simulink model "power_estimator2"  (R2015a)
settings: Solver=ode45  StartTime=0.0  StopTime=10.0  RelTol=1e-3
values from neighbouring files (symbols this model uses):
  L = 8e-3    (= 0.008)    [VOC_param.m]    (also in VOC_param_paper.m = 0.003; controller_parameters.m = 0.003; current_controller_param.m = 0.005; power_control_param.m = 0.01)
settings Model: Creator=rblan  LastModifiedBy=rblan

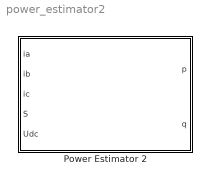
== system power_estimator2 ==
  Power Estimator 2 : Subsystem

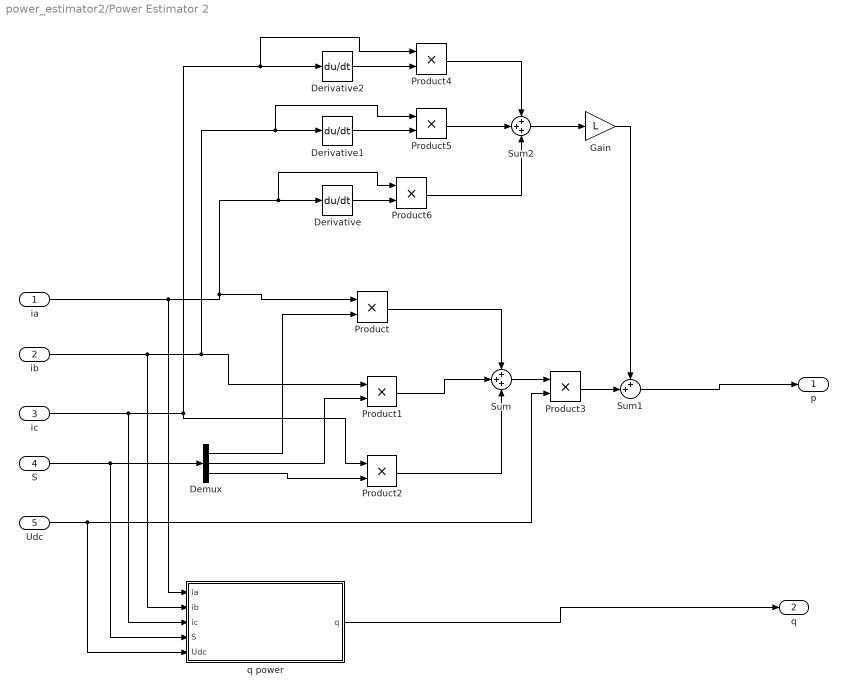
== system power_estimator2/Power Estimator 2 ==
  ia : Inport
  "ib " : Inport  Port=2
  "ic " : Inport  Port=3
  "S " : Inport  Port=4
  Udc : Inport  Port=5
  Demux : Demux  Outputs=3
  Derivative : Derivative
  Derivative1 : Derivative
  Derivative2 : Derivative
  Gain : Gain  Gain=L
  Product{,1..6} (7 alike) : Product
  Sum : Sum  Inputs=+++
  Sum1 : Sum  Inputs=++|
  Sum2 : Sum  Inputs=+++
  "q power " : Subsystem
  p : Outport
  q : Outport  Port=2
  wires:
  "S "/1 -> "q power "/4("S "), Demux/1
  Demux/1 -> Product/2
  ia/1 -> "q power "/1(ia), Product6/1, Derivative/1, Product/1
  "ib "/1 -> "q power "/2("ib "), Product5/1, Derivative1/1, Product1/1
  Demux/2 -> Product1/2
  Demux/3 -> Product2/2
  Product/1 -> Sum/1
  Product1/1 -> Sum/2
  Product2/1 -> Sum/3
  Sum/1 -> Product3/1
  Derivative2/1 -> Product4/2
  Derivative1/1 -> Product5/2
  Derivative/1 -> Product6/2
  Product4/1 -> Sum2/1
  Product5/1 -> Sum2/2
  Product6/1 -> Sum2/3
  Sum2/1 -> Gain/1
  Product3/1 -> Sum1/2
  Gain/1 -> Sum1/1
  "ic "/1 -> "q power "/3("ic "), Product2/1, Product4/1, Derivative2/1
  Udc/1 -> "q power "/5(Udc), Product3/2
  "q power "/1("q ") -> q/1
  Sum1/1 -> p/1

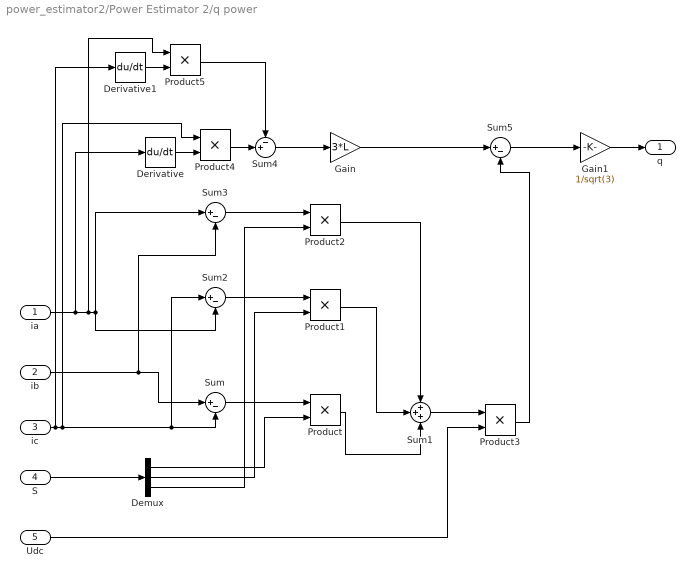
== system power_estimator2/Power Estimator 2/q power  ==
  ia : Inport
  "ib " : Inport  Port=2
  "ic " : Inport  Port=3
  "S " : Inport  Port=4
  Udc : Inport  Port=5
  Demux : Demux  Outputs=3
  Derivative : Derivative
  Derivative1 : Derivative
  Gain : Gain  Gain=3*L
  Gain1 : Gain  Gain=1/sqrt(3)
  Product{,1..5} (6 alike) : Product
  Sum{,2..3,5} (4 alike) : Sum  Inputs=|+-
  Sum1 : Sum  Inputs=+++
  Sum4 : Sum  Inputs=-+|
  "q " : Outport
  wires:
  "ib "/1 -> Sum3/2, Sum/1
  Sum/1 -> Product/1
  "S "/1 -> Demux/1
  Demux/1 -> Product/2
  Sum2/1 -> Product1/1
  Demux/2 -> Product1/2
  Sum3/1 -> Product2/1
  Demux/3 -> Product2/2
  Sum1/1 -> Product3/1
  Udc/1 -> Product3/2
  Derivative/1 -> Product4/2
  ia/1 -> Derivative/1, Product5/1, Sum2/2, Sum3/1
  "ic "/1 -> Derivative1/1, Product4/1, Sum2/1, Sum/2
  Derivative1/1 -> Product5/2
  Product5/1 -> Sum4/1
  Product4/1 -> Sum4/2
  Sum4/1 -> Gain/1
  Gain/1 -> Sum5/1
  Product3/1 -> Sum5/2
  Sum5/1 -> Gain1/1
  Gain1/1 -> "q "/1
  Product2/1 -> Sum1/1
  Product/1 -> Sum1/3
  Product1/1 -> Sum1/2
